simulink model "CM200C_DmaCfgAndUse"  (R2013b)
settings: Solver=ode1  StartTime=0.0  StopTime=Inf  FixedStep=0.001  RelTol=1e-3
libraries: simulink x2
(part 2 of 2)

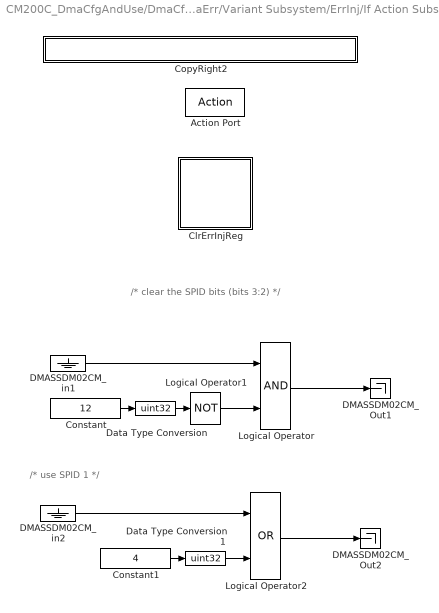
== system CM200C_DmaCfgAndUse/DmaCfgAndUse/InjDmaErr/Variant Subsystem/ErrInj/If Action Subsystem ==
  note: /* use SPID 1 */
  note: /* clear the SPID bits (bits 3:2) */
  Action Port : ActionPort
  ClrErrInjReg : Subsystem
      settings: AttributesFormatString=Client Call : Clear the Fault Injection Register
  Constant : Constant  Value=12  OutDataTypeStr=uint32
  Constant1 : Constant  Value=4  OutDataTypeStr=uint32
  CopyRight2 : Subsystem  Description=|  mask(Copyright Information){none=on}
      | Copyright info block.                                               
      |                                                                     
      | Place copyright information at the top of every subsystem in design.
      mask prompts: none "No parameters"
      mask help: Place copyright information at the top of every subsystem in design.
      mask Display:
      | NxtrConf = 'Nexteer Confidential';
      | 
      | sys = bdroot; %handle for the current model ("system")
      | first = get_param(sys,'Created');
      | first = first(end-3:end);  %year is last four digits
      | 
      | last = get_param(sys,'LastModifiedDate');
      | if isempty(last)
      |     last = datestr(now,'yyyy');
      | else
      |     last = last(end-3:end);
      | end
      | 
      | if strcmp(first,last)
      |     fprintf('%s -- Copyright %s Nexteer',NxtrConf,first)
      | else
      |     fprintf('%s -- %s%s- %s Nexteer',NxtrConf,char(169),first,last)
      | end
  DMASSDM02CM_Out1 : Terminator
  DMASSDM02CM_Out2 : Terminator
  DMASSDM02CM_in1 : Ground
  DMASSDM02CM_in2 : Ground
  Data Type Conversion : DataTypeConversion  OutDataTypeStr=uint32
  Data Type Conversion1 : DataTypeConversion  OutDataTypeStr=uint32
  Logical Operator : Logic  AllPortsSameDT=off  OutDataTypeStr=boolean
  Logical Operator1 : Logic  Operator=NOT  Inputs=1  AllPortsSameDT=off  OutDataTypeStr=boolean
  Logical Operator2 : Logic  Operator=OR  AllPortsSameDT=off  OutDataTypeStr=boolean
  wires:
  Logical Operator/1 -> DMASSDM02CM_Out1/1
  Constant/1 -> Data Type Conversion/1
  Data Type Conversion/1 -> Logical Operator1/1
  Logical Operator1/1 -> Logical Operator/2
  DMASSDM02CM_in1/1 -> Logical Operator/1
  Logical Operator2/1 -> DMASSDM02CM_Out2/1
  Constant1/1 -> Data Type Conversion1/1
  Data Type Conversion1/1 -> Logical Operator2/2
  DMASSDM02CM_in2/1 -> Logical Operator2/1

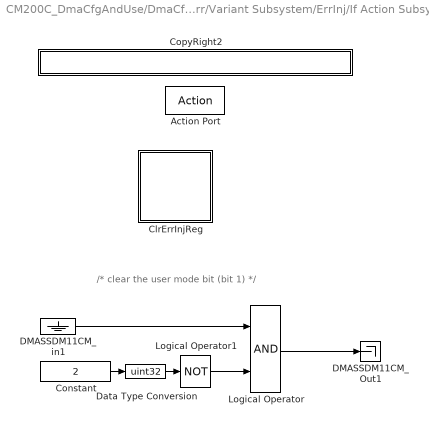
== system CM200C_DmaCfgAndUse/DmaCfgAndUse/InjDmaErr/Variant Subsystem/ErrInj/If Action Subsystem1 ==
  note: /* clear the user mode bit (bit 1) */
  Action Port : ActionPort
  ClrErrInjReg : Subsystem
      settings: AttributesFormatString=Client Call : Clear the Fault Injection Register
  Constant : Constant  Value=2  OutDataTypeStr=uint32
  CopyRight2 : Subsystem  Description=|  mask(Copyright Information){none=on}
      | Copyright info block.                                               
      |                                                                     
      | Place copyright information at the top of every subsystem in design.
      mask prompts: none "No parameters"
      mask help: Place copyright information at the top of every subsystem in design.
      mask Display:
      | NxtrConf = 'Nexteer Confidential';
      | 
      | sys = bdroot; %handle for the current model ("system")
      | first = get_param(sys,'Created');
      | first = first(end-3:end);  %year is last four digits
      | 
      | last = get_param(sys,'LastModifiedDate');
      | if isempty(last)
      |     last = datestr(now,'yyyy');
      | else
      |     last = last(end-3:end);
      | end
      | 
      | if strcmp(first,last)
      |     fprintf('%s -- Copyright %s Nexteer',NxtrConf,first)
      | else
      |     fprintf('%s -- %s%s- %s Nexteer',NxtrConf,char(169),first,last)
      | end
  DMASSDM11CM_Out1 : Terminator
  DMASSDM11CM_in1 : Ground
  Data Type Conversion : DataTypeConversion  OutDataTypeStr=uint32
  Logical Operator : Logic  AllPortsSameDT=off  OutDataTypeStr=boolean
  Logical Operator1 : Logic  Operator=NOT  Inputs=1  AllPortsSameDT=off  OutDataTypeStr=boolean
  wires:
  Logical Operator/1 -> DMASSDM11CM_Out1/1
  Constant/1 -> Data Type Conversion/1
  Data Type Conversion/1 -> Logical Operator1/1
  Logical Operator1/1 -> Logical Operator/2
  DMASSDM11CM_in1/1 -> Logical Operator/1

== system CM200C_DmaCfgAndUse/DmaCfgAndUse/InjDmaErr/Variant Subsystem/ErrInj/If Action Subsystem2 ==
  note: // Modify the ADC0 DMA01 Destination Address  for create data transfer error
      | Disable to Change before configured and Enable the channel.
  Action Port : ActionPort
  ClrErrInjReg : Subsystem
      settings: AttributesFormatString=Client Call : Clear the Fault Injection Register
  CopyRight2 : Subsystem  Description=|  mask(Copyright Information){none=on}
      | Copyright info block.                                               
      |                                                                     
      | Place copyright information at the top of every subsystem in design.
      mask prompts: none "No parameters"
      mask help: Place copyright information at the top of every subsystem in design.
      mask Display:
      | NxtrConf = 'Nexteer Confidential';
      | 
      | sys = bdroot; %handle for the current model ("system")
      | first = get_param(sys,'Created');
      | first = first(end-3:end);  %year is last four digits
      | 
      | last = get_param(sys,'LastModifiedDate');
      | if isempty(last)
      |     last = datestr(now,'yyyy');
      | else
      |     last = last(end-3:end);
      | end
      | 
      | if strcmp(first,last)
      |     fprintf('%s -- Copyright %s Nexteer',NxtrConf,first)
      | else
      |     fprintf('%s -- %s%s- %s Nexteer',NxtrConf,char(169),first,last)
      | end
  DMASSDDA1 : Terminator
  DMASSDRDA1 : Terminator
  FEBFFFFC : Ground
  wires:
  FEBFFFFC/1 -> DMASSDRDA1/1, DMASSDDA1/1

== system CM200C_DmaCfgAndUse/DmaCfgAndUse/InjDmaErr/Variant Subsystem/ErrInj/ReadErrInjReg ==
  CopyRight2 : Subsystem  Description=|  mask(Copyright Information){none=on}
      | Copyright info block.                                               
      |                                                                     
      | Place copyright information at the top of every subsystem in design.
      mask prompts: none "No parameters"
      mask help: Place copyright information at the top of every subsystem in design.
      mask Display:
      | NxtrConf = 'Nexteer Confidential';
      | 
      | sys = bdroot; %handle for the current model ("system")
      | first = get_param(sys,'Created');
      | first = first(end-3:end);  %year is last four digits
      | 
      | last = get_param(sys,'LastModifiedDate');
      | if isempty(last)
      |     last = datestr(now,'yyyy');
      | else
      |     last = last(end-3:end);
      | end
      | 
      | if strcmp(first,last)
      |     fprintf('%s -- Copyright %s Nexteer',NxtrConf,first)
      | else
      |     fprintf('%s -- %s%s- %s Nexteer',NxtrConf,char(169),first,last)
      | end
  Ground : Ground
  ErrId : Outport
  wires:
  Ground/1 -> ErrId/1

== system CM200C_DmaCfgAndUse/DmaCfgAndUse/InjMcuDiagcErr/Variant Subsystem/ErrInj/Action ==
  Action Port : ActionPort
  ClrErrInjReg : Subsystem
      settings: AttributesFormatString=Client Call : Clear the Fault Injection Register
  Constant : Constant  Value=0  OutDataTypeStr=uint32
  CopyRight2 : Subsystem  Description=|  mask(Copyright Information){none=on}
      | Copyright info block.                                               
      |                                                                     
      | Place copyright information at the top of every subsystem in design.
      mask prompts: none "No parameters"
      mask help: Place copyright information at the top of every subsystem in design.
      mask Display:
      | NxtrConf = 'Nexteer Confidential';
      | 
      | sys = bdroot; %handle for the current model ("system")
      | first = get_param(sys,'Created');
      | first = first(end-3:end);  %year is last four digits
      | 
      | last = get_param(sys,'LastModifiedDate');
      | if isempty(last)
      |     last = datestr(now,'yyyy');
      | else
      |     last = last(end-3:end);
      | end
      | 
      | if strcmp(first,last)
      |     fprintf('%s -- Copyright %s Nexteer',NxtrConf,first)
      | else
      |     fprintf('%s -- %s%s- %s Nexteer',NxtrConf,char(169),first,last)
      | end
  DMASSDCEN15_Out1 : Terminator
  wires:
  Constant/1 -> DMASSDCEN15_Out1/1

== system CM200C_DmaCfgAndUse/DmaCfgAndUse/InjMcuDiagcErr/Variant Subsystem/ErrInj/CopyRight2 ==

== system CM200C_DmaCfgAndUse/DmaCfgAndUse/InjMcuDiagcErr/Variant Subsystem/ErrInj/ReadErrInjReg ==
  CopyRight2 : Subsystem  Description=|  mask(Copyright Information){none=on}
      | Copyright info block.                                               
      |                                                                     
      | Place copyright information at the top of every subsystem in design.
      mask prompts: none "No parameters"
      mask help: Place copyright information at the top of every subsystem in design.
      mask Display:
      | NxtrConf = 'Nexteer Confidential';
      | 
      | sys = bdroot; %handle for the current model ("system")
      | first = get_param(sys,'Created');
      | first = first(end-3:end);  %year is last four digits
      | 
      | last = get_param(sys,'LastModifiedDate');
      | if isempty(last)
      |     last = datestr(now,'yyyy');
      | else
      |     last = last(end-3:end);
      | end
      | 
      | if strcmp(first,last)
      |     fprintf('%s -- Copyright %s Nexteer',NxtrConf,first)
      | else
      |     fprintf('%s -- %s%s- %s Nexteer',NxtrConf,char(169),first,last)
      | end
  Ground : Ground
  ErrId : Outport
  wires:
  Ground/1 -> ErrId/1

== system CM200C_DmaCfgAndUse/DmaCfgAndUse/DmaEna2MilliSecToMotCtrlTrf/Variant Subsystem/ErrInj/If Action Subsystem/CopyRight2 ==

== system CM200C_DmaCfgAndUse/DmaCfgAndUse/DmaEna2MilliSecToMotCtrlTrf/Variant Subsystem/ErrInj/ReadErrInjReg/CopyRight2 ==

== system CM200C_DmaCfgAndUse/DmaCfgAndUse/InjDmaErr/Variant Subsystem/ErrInj/If Action Subsystem/ClrErrInjReg ==
  CopyRight2 : Subsystem  Description=|  mask(Copyright Information){none=on}
      | Copyright info block.                                               
      |                                                                     
      | Place copyright information at the top of every subsystem in design.
      mask prompts: none "No parameters"
      mask help: Place copyright information at the top of every subsystem in design.
      mask Display:
      | NxtrConf = 'Nexteer Confidential';
      | 
      | sys = bdroot; %handle for the current model ("system")
      | first = get_param(sys,'Created');
      | first = first(end-3:end);  %year is last four digits
      | 
      | last = get_param(sys,'LastModifiedDate');
      | if isempty(last)
      |     last = datestr(now,'yyyy');
      | else
      |     last = last(end-3:end);
      | end
      | 
      | if strcmp(first,last)
      |     fprintf('%s -- Copyright %s Nexteer',NxtrConf,first)
      | else
      |     fprintf('%s -- %s%s- %s Nexteer',NxtrConf,char(169),first,last)
      | end

== system CM200C_DmaCfgAndUse/DmaCfgAndUse/InjDmaErr/Variant Subsystem/ErrInj/If Action Subsystem/CopyRight2 ==

== system CM200C_DmaCfgAndUse/DmaCfgAndUse/InjDmaErr/Variant Subsystem/ErrInj/If Action Subsystem1/ClrErrInjReg ==
  CopyRight2 : Subsystem  Description=|  mask(Copyright Information){none=on}
      | Copyright info block.                                               
      |                                                                     
      | Place copyright information at the top of every subsystem in design.
      mask prompts: none "No parameters"
      mask help: Place copyright information at the top of every subsystem in design.
      mask Display:
      | NxtrConf = 'Nexteer Confidential';
      | 
      | sys = bdroot; %handle for the current model ("system")
      | first = get_param(sys,'Created');
      | first = first(end-3:end);  %year is last four digits
      | 
      | last = get_param(sys,'LastModifiedDate');
      | if isempty(last)
      |     last = datestr(now,'yyyy');
      | else
      |     last = last(end-3:end);
      | end
      | 
      | if strcmp(first,last)
      |     fprintf('%s -- Copyright %s Nexteer',NxtrConf,first)
      | else
      |     fprintf('%s -- %s%s- %s Nexteer',NxtrConf,char(169),first,last)
      | end

== system CM200C_DmaCfgAndUse/DmaCfgAndUse/InjDmaErr/Variant Subsystem/ErrInj/If Action Subsystem1/CopyRight2 ==

== system CM200C_DmaCfgAndUse/DmaCfgAndUse/InjDmaErr/Variant Subsystem/ErrInj/If Action Subsystem2/ClrErrInjReg ==
  CopyRight2 : Subsystem  Description=|  mask(Copyright Information){none=on}
      | Copyright info block.                                               
      |                                                                     
      | Place copyright information at the top of every subsystem in design.
      mask prompts: none "No parameters"
      mask help: Place copyright information at the top of every subsystem in design.
      mask Display:
      | NxtrConf = 'Nexteer Confidential';
      | 
      | sys = bdroot; %handle for the current model ("system")
      | first = get_param(sys,'Created');
      | first = first(end-3:end);  %year is last four digits
      | 
      | last = get_param(sys,'LastModifiedDate');
      | if isempty(last)
      |     last = datestr(now,'yyyy');
      | else
      |     last = last(end-3:end);
      | end
      | 
      | if strcmp(first,last)
      |     fprintf('%s -- Copyright %s Nexteer',NxtrConf,first)
      | else
      |     fprintf('%s -- %s%s- %s Nexteer',NxtrConf,char(169),first,last)
      | end

== system CM200C_DmaCfgAndUse/DmaCfgAndUse/InjDmaErr/Variant Subsystem/ErrInj/If Action Subsystem2/CopyRight2 ==

== system CM200C_DmaCfgAndUse/DmaCfgAndUse/InjDmaErr/Variant Subsystem/ErrInj/ReadErrInjReg/CopyRight2 ==

== system CM200C_DmaCfgAndUse/DmaCfgAndUse/InjMcuDiagcErr/Variant Subsystem/ErrInj/Action/ClrErrInjReg ==
  CopyRight2 : Subsystem  Description=|  mask(Copyright Information){none=on}
      | Copyright info block.                                               
      |                                                                     
      | Place copyright information at the top of every subsystem in design.
      mask prompts: none "No parameters"
      mask help: Place copyright information at the top of every subsystem in design.
      mask Display:
      | NxtrConf = 'Nexteer Confidential';
      | 
      | sys = bdroot; %handle for the current model ("system")
      | first = get_param(sys,'Created');
      | first = first(end-3:end);  %year is last four digits
      | 
      | last = get_param(sys,'LastModifiedDate');
      | if isempty(last)
      |     last = datestr(now,'yyyy');
      | else
      |     last = last(end-3:end);
      | end
      | 
      | if strcmp(first,last)
      |     fprintf('%s -- Copyright %s Nexteer',NxtrConf,first)
      | else
      |     fprintf('%s -- %s%s- %s Nexteer',NxtrConf,char(169),first,last)
      | end

== system CM200C_DmaCfgAndUse/DmaCfgAndUse/InjMcuDiagcErr/Variant Subsystem/ErrInj/Action/CopyRight2 ==

== system CM200C_DmaCfgAndUse/DmaCfgAndUse/InjMcuDiagcErr/Variant Subsystem/ErrInj/ReadErrInjReg/CopyRight2 ==

== system CM200C_DmaCfgAndUse/DmaCfgAndUse/InjDmaErr/Variant Subsystem/ErrInj/If Action Subsystem/ClrErrInjReg/CopyRight2 ==

== system CM200C_DmaCfgAndUse/DmaCfgAndUse/InjDmaErr/Variant Subsystem/ErrInj/If Action Subsystem1/ClrErrInjReg/CopyRight2 ==

== system CM200C_DmaCfgAndUse/DmaCfgAndUse/InjDmaErr/Variant Subsystem/ErrInj/If Action Subsystem2/ClrErrInjReg/CopyRight2 ==

== system CM200C_DmaCfgAndUse/DmaCfgAndUse/InjMcuDiagcErr/Variant Subsystem/ErrInj/Action/ClrErrInjReg/CopyRight2 ==
